simulink model "ZT_VehCtrl_18B"  (R2018b)
settings: Solver=FixedStepAuto  StartTime=0.0  StopTime=inf  FixedStep=0.005  RelTol=1e-3
InitFcn:
  | mbd_mpc_consistency_checks(bdroot(gcs));
undefined symbols (not defined in the file): ANG_DEAD, BMS_NormalPwr, BrkPrsByBrkPct_TB_X, BrkPrsByBrkPct_TB_Y, DELAY_DISCHARGE, DELAY_RCUOFF, DRV_BACKWARD, DRV_BRAKE, DRV_FORWARD, DRV_NEUTRAL, DRV_PARK, DRV_UNPARK, DRV_ZEROTURN, EPB_LOCK, EPB_UNLOCK, ExtraLoadPwr, FanOff, fifo_0_vect, fifo_1_vect, HiFanReq, HV_finished, HV_No_Active, HV_POWER_OFF, HV_POWER_ON, HVDown, HVON, KaTLS_v_DrgUp_X_VehSpd, KeFTM_s_Way1OffDlyTime, KeFTM_TK_Way1CoolLv2OffBatTemp, KeFTM_TK_Way1CoolLv2OffMtrTemp, KeFTM_TK_Way1CoolLv2OnBatTemp, KeFTM_TK_Way1CoolLv2OnMtrTemp, KeFTM_TK_Way1CoolLv3OffBatTemp, KeFTM_TK_Way1CoolLv3OffMtrTemp, KeFTM_TK_Way1CoolLv3OnBatTemp, KeFTM_TK_Way1CoolLv3OnMtrTemp, KeFTM_TK_Way1CoolLv4OffBatTemp, KeFTM_TK_Way1CoolLv4OffMtrTemp, KeFTM_TK_Way1CoolLv4OnBatTemp, KeFTM_TK_Way1CoolLv4OnMtrTemp, Kp1, Kp2, LowFanReq, LQFP, MtrPwrFactor_RCU, MtrPwrHighToMidThd, MtrPwrLowToMidThd, MtrPwrMidToHighThd, MtrPwrMidToLowThd, MtrTrqMax, PCT_DEAD, Precharge, PTO_1000, PTO_540, pts1_fifo_0_vect, pts1_fifo_1_vect, pts2_fifo_0_vect, pts2_fifo_1_vect, pts3_fifo_0_vect, pts3_fifo_1_vect ... (+24)
libraries: mbd_mpc574x_ec_toolbox x124, canmsglib x72, simulink x57
(part 3 of 11)

== system ZT_VehCtrl_18B/SigIn/PWM ==
  note: DI PWM PULLDOWN
  note: DI PWM PULLUP
  Bus Creator : BusCreator  Inputs=8
  Data Store Read : DataStoreRead  DataStoreName=DI31_PWM_DC
  Data Store Read1 : DataStoreRead  DataStoreName=DI31_PWM_FRQ
  Data Store Read2 : DataStoreRead  DataStoreName=DI32_PWM_DC
  Data Store Read3 : DataStoreRead  DataStoreName=DI32_PWM_FRQ
  Data Store Read4 : DataStoreRead  DataStoreName=DI33_PWM_DC
  Data Store Read5 : DataStoreRead  DataStoreName=DI33_PWM_FRQ
  Data Store Read6 : DataStoreRead  DataStoreName=DI34_PWM_DC
  Data Store Read7 : DataStoreRead  DataStoreName=DI34_PWM_FRQ
  Data Store Write : DataStoreWrite  DataStoreName=DI31_PWM_DC
  Data Store Write1 : DataStoreWrite  DataStoreName=DI31_PWM_FRQ
  Data Store Write2 : DataStoreWrite  DataStoreName=DI32_PWM_DC
  Data Store Write3 : DataStoreWrite  DataStoreName=DI32_PWM_FRQ
  Data Store Write4 : DataStoreWrite  DataStoreName=DI33_PWM_DC
  Data Store Write5 : DataStoreWrite  DataStoreName=DI33_PWM_FRQ
  Data Store Write6 : DataStoreWrite  DataStoreName=DI34_PWM_FRQ
  Data Store Write7 : DataStoreWrite  DataStoreName=DI34_PWM_DC
  PWM_PTS1 : Subsystem
  PWM_PTS2 : Subsystem
  PWM_PTS3 : Subsystem
  PWM_PTS4 : Subsystem
  Subsystem : Subsystem  Commented=on
  eTimer_Arm_Capture : mbd_mpc574x_ec_toolbox/Motor Control Blocks/eTIMER Blocks/eTimer_Arm_Capture  etimerModule=0  etimerChannel=2  etimerArmAction=Start
  eTimer_Arm_Capture1 : mbd_mpc574x_ec_toolbox/Motor Control Blocks/eTIMER Blocks/eTimer_Arm_Capture  etimerModule=1  etimerChannel=2  etimerArmAction=Start
  eTimer_Arm_Capture2 : mbd_mpc574x_ec_toolbox/Motor Control Blocks/eTIMER Blocks/eTimer_Arm_Capture  etimerModule=1  etimerChannel=1  etimerArmAction=Start
  eTimer_Arm_Capture3 : mbd_mpc574x_ec_toolbox/Motor Control Blocks/eTIMER Blocks/eTimer_Arm_Capture  etimerModule=1  etimerChannel=3  etimerArmAction=Start
  PWMIn : Outport
  wires:
  Bus Creator/1 -> PWMIn/1
  Data Store Read7/1 -> Bus Creator/8  "DI34_PWM_FRQ"
  Data Store Read6/1 -> Bus Creator/7  "DI34_PWM_DC"
  Data Store Read5/1 -> Bus Creator/6  "DI33_PWM_FRQ"
  Data Store Read4/1 -> Bus Creator/5  "DI33_PWM_DC"
  Data Store Read3/1 -> Bus Creator/4  "DI32_PWM_FRQ"
  Data Store Read2/1 -> Bus Creator/3  "DI32_PWM_DC"
  Data Store Read1/1 -> Bus Creator/2  "DI31_PWM_FRQ"
  Data Store Read/1 -> Bus Creator/1  "DI31_PWM_DC"
  PWM_PTS4/1(DC) -> Data Store Write/1
  PWM_PTS4/2(freq) -> Data Store Write1/1
  PWM_PTS1/1(DC) -> Data Store Write2/1
  PWM_PTS1/2(freq) -> Data Store Write3/1
  PWM_PTS2/1(DC) -> Data Store Write4/1
  PWM_PTS2/2(freq) -> Data Store Write5/1
  PWM_PTS3/2(freq) -> Data Store Write6/1
  PWM_PTS3/1(DC) -> Data Store Write7/1

== system ZT_VehCtrl_18B/SigOut/ACU ==
  "ACU_OUT " : Inport
  Trigger : TriggerPort  VariantControl=Variant  PortDimensions=1
  Bus Selector : BusSelector  OutputSignals=Data,Length
  FCAN_Send_ID_0x0C079AA7 : mbd_mpc574x_ec_toolbox/Communication Blocks/CAN Blocks/FCAN_Send  Priority=2  can_instance=1  can_mode=Non-blocking  can_timeout_ms=0  can_mb_idx=43  can_extended_id=on  can_is_remote=off  can_id=0C079AA7  show_adv_opts=off  can_fd_enable=off  can_enable_brs=off  can_fd_padding=0
      settings: SourceProductName=NXP Model-Based Design Toolbox for MPC57xx MCUs
  VCU_ACU1 : canmsglib/CAN Pack  CANdbFile=D:\VCU\VCU_SL_ZhengZhou\ZT2\模型与接口\CAN_DBC\动力CANB_GBK.dbc  MsgList=VCU_ACU1  MsgName=VCU_ACU1  MsgIDType=Extended (29-bit identifier)  MsgIdentifier=201824935  MsgLength=8  SignalInfo=DcacAcCmd$32$8$1$2$1$0$1$0$-Inf$Inf$#DcacEpsCmd$16$8$1$2$1$0$1$0$-Inf$Inf$#DcacEpsMode$24$8$1$2$1$0$1$0$-Inf$Inf$#DcdcCmd$0$8$1$2$1$0$1$0$-Inf$Inf$#  NSignals=4  StartBits=str2num('[int32(32);int32(16);int32(24);int32(0)]')  SignalSizes=str2num('[int32(8);int32(8);int32(8);int32(8)]')  ByteOrders=str2num('[int32(1);int32(1);int32(1);int32(1)]')  DataTypes=str2num('[int32(2);int32(2);int32(2);int32(2)]')  MultiplexTypes=str2num('[int32(1);int32(1);int32(1);int32(1)]')  MultiplexValues=str2num('[double(0);double(0);double(0);double(0)]')  Factors=str2num('[double(1);double(1);double(1);double(1)]')  Offsets=str2num('[double(0);double(0);double(0);double(0)]')  Minimums=str2num('[double(-Inf);double(-Inf);double(-Inf);double(-Inf)]')  Maximums=str2num('[double(Inf);double(Inf);double(Inf);double(Inf)]')  Remote=off  ApplyMinMax=off  BusOutput=on
      settings: SourceProductName=Simulink Real-Time  SourceProductBaseCode=XP  DataFormat=CANdb specified signals
  wires:
  VCU_ACU1/1 -> Bus Selector/1
  Bus Selector/2 -> FCAN_Send_ID_0x0C079AA7/2  "<Length>"
  Bus Selector/1 -> FCAN_Send_ID_0x0C079AA7/1  "<Data>"

== system ZT_VehCtrl_18B/SigOut/BMS ==
  "BMS_OUT " : Inport
  Trigger : TriggerPort  VariantControl=Variant  PortDimensions=1
  Bus Selector : BusSelector  OutputSignals=Data,Length
  FCAN_Send_ID_0x160 : mbd_mpc574x_ec_toolbox/Communication Blocks/CAN Blocks/FCAN_Send  Priority=2  can_instance=0  can_mode=Non-blocking  can_timeout_ms=0  can_mb_idx=43  can_extended_id=off  can_is_remote=off  can_id=160  show_adv_opts=off  can_fd_enable=off  can_enable_brs=off  can_fd_padding=0
      settings: SourceProductName=NXP Model-Based Design Toolbox for MPC57xx MCUs
  VCU_BMS : canmsglib/CAN Pack  CANdbFile=D:\VCU\VCU_SL_ZhengZhou\ZT2\模型与接口\CAN_DBC\整车CANA_GBK.dbc  MsgList=VCU_BMS  MsgName=VCU_BMS  MsgIDType=Standard (11-bit identifier)  MsgIdentifier=352  MsgLength=8  SignalInfo=VCU_PowerOnReq$0$1$2$2$1$0$1$0$0$1$#VCU_UrgencyCutOffPowerReq$1$1$2$2$1$0$1$0$0$1$#  NSignals=2  StartBits=str2num('[int32(0);int32(1)]')  SignalSizes=str2num('[int32(1);int32(1)]')  ByteOrders=str2num('[int32(2);int32(2)]')  DataTypes=str2num('[int32(2);int32(2)]')  MultiplexTypes=str2num('[int32(1);int32(1)]')  MultiplexValues=str2num('[double(0);double(0)]')  Factors=str2num('[double(1);double(1)]')  Offsets=str2num('[double(0);double(0)]')  Minimums=str2num('[double(0);double(0)]')  Maximums=str2num('[double(1);double(1)]')  Remote=off  ApplyMinMax=off  BusOutput=on
      settings: SourceProductName=Simulink Real-Time  SourceProductBaseCode=XP  DataFormat=CANdb specified signals
  wires:
  VCU_BMS/1 -> Bus Selector/1
  Bus Selector/2 -> FCAN_Send_ID_0x160/2  "<Length>"
  Bus Selector/1 -> FCAN_Send_ID_0x160/1  "<Data>"

== system ZT_VehCtrl_18B/SigOut/BRS ==
  "BRS_OUT " : Inport
  Trigger : TriggerPort  VariantControl=Variant  PortDimensions=1
  Bus Selector : BusSelector  OutputSignals=Data,Length
  Bus Selector1 : BusSelector  OutputSignals=DCDC_Enable
  FCAN_Send_ID_0x0CF109A7 : mbd_mpc574x_ec_toolbox/Communication Blocks/CAN Blocks/FCAN_Send  Priority=2  can_instance=0  can_mode=Non-blocking  can_timeout_ms=0  can_mb_idx=44  can_extended_id=on  can_is_remote=off  can_id=0CF109A7  show_adv_opts=off  can_fd_enable=off  can_enable_brs=off  can_fd_padding=0
      settings: SourceProductName=NXP Model-Based Design Toolbox for MPC57xx MCUs
  VCU2BRS : canmsglib/CAN Pack  CANdbFile=D:\VCU\VCU_SL_ZhengZhou\ZT2\模型与接口\CAN_DBC\整车CANA_GBK.dbc  MsgList=VCU2BRS  MsgName=VCU2BRS  MsgIDType=Extended (29-bit identifier)  MsgIdentifier=217123239  MsgLength=8  SignalInfo=LiveCounter$56$8$1$2$1$0$1$0$0$255$#MaxChargePowerLimit$16$16$1$2$1$0$1$0$0$500$#OnOffCmd$46$1$1$2$1$0$1$0$0$1$#PowerReq$0$16$1$2$1$0$1$0$0$500$#  NSignals=4  StartBits=str2num('[int32(56);int32(16);int32(46);int32(0)]')  SignalSizes=str2num('[int32(8);int32(16);int32(1);int32(16)]')  ByteOrders=str2num('[int32(1);int32(1);int32(1);int32(1)]')  DataTypes=str2num('[int32(2);int32(2);int32(2);int32(2)]')  MultiplexTypes=str2num('[int32(1);int32(1);int32(1);int32(1)]')  MultiplexValues=str2num('[double(0);double(0);double(0);double(0)]')  Factors=str2num('[double(1);double(1);double(1);double(1)]')  Offsets=str2num('[double(0);double(0);double(0);double(0)]')  Minimums=str2num('[double(0);double(0);double(0);double(0)]')  Maximums=str2num('[double(255);double(500);double(1);double(500)]')  Remote=off  ApplyMinMax=off  BusOutput=on
      settings: SourceProductName=Simulink Real-Time  SourceProductBaseCode=XP  DataFormat=CANdb specified signals
  wires:
  VCU2BRS/1 -> Bus Selector/1
  "BRS_OUT "/1 -> Bus Selector1/1
  Bus Selector/1 -> FCAN_Send_ID_0x0CF109A7/1  "<Data>"
  Bus Selector/2 -> FCAN_Send_ID_0x0CF109A7/2  "<Length>"

== system ZT_VehCtrl_18B/SigOut/DCDC ==
  "DCDC_OUT " : Inport
  Trigger : TriggerPort  VariantControl=Variant  PortDimensions=1
  Bus Selector : BusSelector  OutputSignals=Data,Length
  FCAN_Send_ID_0x18008FD0 : mbd_mpc574x_ec_toolbox/Communication Blocks/CAN Blocks/FCAN_Send  Priority=2  can_instance=1  can_mode=Non-blocking  can_timeout_ms=0  can_mb_idx=43  can_extended_id=on  can_is_remote=off  can_id=18008FD0  show_adv_opts=off  can_fd_enable=off  can_enable_brs=off  can_fd_padding=0
      settings: SourceProductName=NXP Model-Based Design Toolbox for MPC57xx MCUs
  VCU_DCDC1 : canmsglib/CAN Pack  CANdbFile=D:\VCU\VCU_SL_ZhengZhou\ZT2\模型与接口\CAN_DBC\动力CANB_GBK.dbc  MsgList=VCU_DCDC1  MsgName=VCU_DCDC1  MsgIDType=Extended (29-bit identifier)  MsgIdentifier=402690000  MsgLength=8  SignalInfo=VCU_DCDC1_En$0$2$1$2$1$0$1$0$0$3$#  NSignals=1  StartBits=str2num('[int32(0)]')  SignalSizes=str2num('[int32(2)]')  ByteOrders=str2num('[int32(1)]')  DataTypes=str2num('[int32(2)]')  MultiplexTypes=str2num('[int32(1)]')  MultiplexValues=str2num('[double(0)]')  Factors=str2num('[double(1)]')  Offsets=str2num('[double(0)]')  Minimums=str2num('[double(0)]')  Maximums=str2num('[double(3)]')  Remote=off  ApplyMinMax=off  BusOutput=on
      settings: SourceProductName=Simulink Real-Time  SourceProductBaseCode=XP  DataFormat=CANdb specified signals
  wires:
  VCU_DCDC1/1 -> Bus Selector/1
  Bus Selector/2 -> FCAN_Send_ID_0x18008FD0/2  "<Length>"
  Bus Selector/1 -> FCAN_Send_ID_0x18008FD0/1  "<Data>"

== system ZT_VehCtrl_18B/SigOut/GPIO  ==
  note: LS
  note: PWM
  note: HS
  ETC : Subsystem
  HS : Subsystem
  PWM_OUT : Subsystem  Commented=on
  SPI0: LS09_14_15_16_1_2_11_4 : Subsystem
  SPI3: LS03_06_07_08_10_12_13_17_18_19 : Subsystem

== system ZT_VehCtrl_18B/SigOut/HVC ==
  "HVC_OUT " : Inport
  Trigger : TriggerPort  VariantControl=Variant  PortDimensions=1
  Bus Selector : BusSelector  OutputSignals=Data,Length
  Ctrl_HVC : canmsglib/CAN Pack  CANdbFile=D:\VCU\VCU_SL_ZhengZhou\ZT2\模型与接口\CAN_DBC\动力CANB_GBK.dbc  MsgList=Ctrl_HVC  MsgName=Ctrl_HVC  MsgIDType=Extended (29-bit identifier)  MsgIdentifier=402694405  MsgLength=8  SignalInfo=EDrv1_PowOnCmd$0$1$1$2$1$0$1$0$0$1$#EDrv2_PowOnCmd$2$1$1$2$1$0$1$0$0$1$#HvcCmd_Life$60$4$1$2$1$0$1$0$0$15$#PTC_PowOnCmd$6$1$1$2$1$0$1$0$0$1$#PaxAC_PowOnCmd$4$1$1$2$1$0$1$0$0$1$#  NSignals=5  StartBits=str2num('[int32(0);int32(2);int32(60);int32(6);int32(4)]')  SignalSizes=str2num('[int32(1);int32(1);int32(4);int32(1);int32(1)]')  ByteOrders=str2num('[int32(1);int32(1);int32(1);int32(1);int32(1)]')  DataTypes=str2num('[int32(2);int32(2);int32(2);int32(2);int32(2)]')  MultiplexTypes=str2num('[int32(1);int32(1);int32(1);int32(1);int32(1)]')  MultiplexValues=str2num('[double(0);double(0);double(0);double(0);double(0)]')  Factors=str2num('[double(1);double(1);double(1);double(1);double(1)]')  Offsets=str2num('[double(0);double(0);double(0);double(0);double(0)]')  Minimums=str2num('[double(0);double(0);double(0);double(0);double(0)]')  Maximums=str2num('[double(1);double(1);double(15);double(1);double(1)]')  Remote=off  ApplyMinMax=off  BusOutput=on
      settings: SourceProductName=Simulink Real-Time  SourceProductBaseCode=XP  DataFormat=CANdb specified signals
  FCAN_Send_ID_0x1800A105 : mbd_mpc574x_ec_toolbox/Communication Blocks/CAN Blocks/FCAN_Send  Priority=2  can_instance=1  can_mode=Non-blocking  can_timeout_ms=0  can_mb_idx=43  can_extended_id=on  can_is_remote=off  can_id=1800A105  show_adv_opts=off  can_fd_enable=off  can_enable_brs=off  can_fd_padding=0
      settings: SourceProductName=NXP Model-Based Design Toolbox for MPC57xx MCUs
  wires:
  Bus Selector/1 -> FCAN_Send_ID_0x1800A105/1  "<Data>"
  Bus Selector/2 -> FCAN_Send_ID_0x1800A105/2  "<Length>"
  Ctrl_HVC/1 -> Bus Selector/1

== system ZT_VehCtrl_18B/SigOut/ICU1  ==
  "ICU_OUT " : Inport
  Trigger : TriggerPort  VariantControl=Variant  PortDimensions=1
  Bus Selector{,3..7} (6 alike) : BusSelector  OutputSignals=Data,Length
  Bus Selector1 : BusSelector  OutputSignals=DCDC_Enable
  FCAN_Send_ID_0x180128D0 : mbd_mpc574x_ec_toolbox/Communication Blocks/CAN Blocks/FCAN_Send  Priority=2  can_instance=0  can_mode=Non-blocking  can_timeout_ms=0  can_mb_idx=44  can_extended_id=on  can_is_remote=off  can_id=180128D0  show_adv_opts=off  can_fd_enable=off  can_enable_brs=off  can_fd_padding=0
      settings: SourceProductName=NXP Model-Based Design Toolbox for MPC57xx MCUs
  FCAN_Send_ID_0x180328D0 : mbd_mpc574x_ec_toolbox/Communication Blocks/CAN Blocks/FCAN_Send  Priority=2  can_instance=0  can_mode=Non-blocking  can_timeout_ms=0  can_mb_idx=44  can_extended_id=on  can_is_remote=off  can_id=180328D0  show_adv_opts=off  can_fd_enable=off  can_enable_brs=off  can_fd_padding=0
      settings: SourceProductName=NXP Model-Based Design Toolbox for MPC57xx MCUs
  FCAN_Send_ID_0x181128D0 : mbd_mpc574x_ec_toolbox/Communication Blocks/CAN Blocks/FCAN_Send  Priority=2  can_instance=0  can_mode=Non-blocking  can_timeout_ms=0  can_mb_idx=44  can_extended_id=on  can_is_remote=off  can_id=181128D0  show_adv_opts=off  can_fd_enable=off  can_enable_brs=off  can_fd_padding=0
      settings: SourceProductName=NXP Model-Based Design Toolbox for MPC57xx MCUs
  FCAN_Send_ID_0x181228D0 : mbd_mpc574x_ec_toolbox/Communication Blocks/CAN Blocks/FCAN_Send  Priority=2  can_instance=0  can_mode=Non-blocking  can_timeout_ms=0  can_mb_idx=44  can_extended_id=on  can_is_remote=off  can_id=181228D0  show_adv_opts=off  can_fd_enable=off  can_enable_brs=off  can_fd_padding=0
      settings: SourceProductName=NXP Model-Based Design Toolbox for MPC57xx MCUs
  FCAN_Send_ID_0x181328D0 : mbd_mpc574x_ec_toolbox/Communication Blocks/CAN Blocks/FCAN_Send  Priority=2  can_instance=1  can_mode=Non-blocking  can_timeout_ms=0  can_mb_idx=44  can_extended_id=on  can_is_remote=off  can_id=181328D0  show_adv_opts=off  can_fd_enable=off  can_enable_brs=off  can_fd_padding=0
      settings: SourceProductName=NXP Model-Based Design Toolbox for MPC57xx MCUs
  FCAN_Send_ID_0x181428D0 : mbd_mpc574x_ec_toolbox/Communication Blocks/CAN Blocks/FCAN_Send  Priority=2  can_instance=1  can_mode=Non-blocking  can_timeout_ms=0  can_mb_idx=44  can_extended_id=on  can_is_remote=off  can_id=181428D0  show_adv_opts=off  can_fd_enable=off  can_enable_brs=off  can_fd_padding=0
      settings: SourceProductName=NXP Model-Based Design Toolbox for MPC57xx MCUs
  VCU2MCU1_1 : canmsglib/CAN Pack  CANdbFile=D:\VCU\VCU_SL_ZhengZhou\ZT2\模型与接口\CAN_DBC\整车CANA_GBK.dbc  MsgList=VCU2ICUInfor1  MsgName=VCU2ICUInfor1  MsgIDType=Extended (29-bit identifier)  MsgIdentifier=402729168  MsgLength=8  SignalInfo=VCU_BattSOC_pct$16$8$1$2$1$0$1$0$0$100$#VCU_BattTempHi_b$32$1$1$2$1$0$1$0$0$1$#VCU_BrakeFlt_b$39$1$1$2$1$0$1$0$0$1$#VCU_CoolFanWrkIdc_b$44$1$1$2$1$0$1$0$0$1$#VCU_CoolSysFanPWM$56$8$1$2$1$0$1$0$0$100$#VCU_CoolSysFltIdc_b$43$1$1$2$1$0$1$0$0$1$#VCU_EmrPumpSt_enum$5$2$1$2$1$0$1$0$0$3$#VCU_FltSt_enum$6$1$1$2$1$0$1$0$0$1$#VCU_GearSt_enum$24$8$1$2$1$0$1$0$0$5$#VCU_HeadLight_b$46$1$1$2$1$0$1$0$0$1$#VCU_HydSysFlt_b$33$1$1$2$1$0$1$0$0$1$#VCU_LShift_b$3$1$1$2$1$0$1$0$0$1$#VCU_MCUTempHiFlt_b$35$1$1$2$1$0$1$0$0$1$#VCU_MtTempHiFlt_b$36$1$1$2$1$0$1$0$0$1$#VCU_Pst_b$0$1$1$2$1$0$1$0$0$1$#VCU_RShift_b$2$1$1$2$1$0$1$0$0$1$#VCU_RearLight_b$45$1$1$2$1$0$1$0$0$1$#VCU_SOCLoFlt_b$1$1$1$2$1$0$1$0$0$1$#VCU_SysWorkStCode_num$48$8$1$2$1$0$1$0$0$255$#VCU_TopWrkSt_b$38$1$1$2$1$0$1$0$0$1$#VCU_VehACharge_b$34$1$1$2$1$0$1$0$0$1$#VCU_VehDCharge_b$37$1$1$2$1$0$1$0$0$1$#VCU_VehSpd_kmh$8$8$1$2$1$0$1$0$0$255$#VCU_WatPumpOpenSt_b$47$1$1$2$1$0$1$0$0$1$#VCU_WrkSt_enum$7$1$1$2$1$0$1$0$0$1$#  NSignals=25  StartBits=str2num('[int32(16);int32(32);int32(39);int32(44);int32(56);int32(43);int32(5);int32(6);int32(24);int32(46);int32(33);int32(3);int32(35);int32(36);int32(0);int32(2);int32(45);int32(1);int32(48);int32(38);int32(34);int32(37);int32(8);int32(47);int32(7)]')  SignalSizes=str2num('[int32(8);int32(1);int32(1);int32(1);int32(8);int32(1);int32(2);int32(1);int32(8);int32(1);int32(1);int32(1);int32(1);int32(1);int32(1);int32(1);int32(1);int32(1);int32(8);int32(1);int32(1);int32(1);int32(8);int32(1);int32(1)]')  ByteOrders=str2num('[int32(1);int32(1);int32(1);int32(1);int32(1);int32(1);int32(1);int32(1);int32(1);int32(1);int32(1);int32(1);int32(1);int32(1);int32(1);int32(1);int32(1);int32(1);int32(1);int32(1);int32(1);int32(1);int32(1);int32(1);int32(1)]')  DataTypes=str2num('[int32(2);int32(2);int32(2);int32(2);int32(2);int32(2);int32(2);int32(2);int32(2);int32(2);int32(2);int32(2);int32(2);int32(2);int32(2);int32(2);int32(2);int32(2);int32(2);int32(2);int32(2);int32(2);int32(2);int32(2);int32(2)]')  MultiplexTypes=str2num('[int32(1);int32(1);int32(1);int32(1);int32(1);int32(1);int32(1);int32(1);int32(1);int32(1);int32(1);int32(1);int32(1);int32(1);int32(1);int32(1);int32(1);int32(1);int32(1);int32(1);int32(1);int32(1);int32(1);int32(1);int32(1)]')  MultiplexValues=str2num('[double(0);double(0);double(0);double(0);double(0);double(0);double(0);double(0);double(0);double(0);double(0);double(0);double(0);double(0);double(0);double(0);double(0);double(0);double(0);double(0);double(0);double(0);double(0);double(0);double(0)]')  Factors=str2num('[double(1);double(1);double(1);double(1);double(1);double(1);double(1);double(1);double(1);double(1);double(1);double(1);double(1);double(1);double(1);double(1);double(1);double(1);double(1);double(1);double(1);double(1);double(1);double(1);double(1)]')  Offsets=str2num('[double(0);double(0);double(0);double(0);double(0);double(0);double(0);double(0);double(0);double(0);double(0);double(0);double(0);double(0);double(0);double(0);double(0);double(0);double(0);double(0);double(0);double(0);double(0);double(0);double(0)]')  Minimums=str2num('[double(0);double(0);double(0);double(0);double(0);double(0);double(0);double(0);double(0);double(0);double(0);double(0);double(0);double(0);double(0);double(0);double(0);double(0);double(0);double(0);double(0);double(0);double(0);double(0);double(0)]')  Maximums=str2num('[double(100);double(1);double(1);double(1);double(100);double(1);double(3);double(1);double(5);double(1);double(1);double(1);double(1);double(1);double(1);double(1);double(1);double(1);double(255);double(1);double(1);double(1);double(255);double(1);double(1)]')  Remote=off  ApplyMinMax=off  BusOutput=on
      settings: SourceProductName=Simulink Real-Time  SourceProductBaseCode=XP  DataFormat=CANdb specified signals
  VCU2MCU1_3 : canmsglib/CAN Pack  CANdbFile=D:\VCU\VCU_SL_ZhengZhou\ZT2\模型与接口\CAN_DBC\整车CANA_GBK.dbc  MsgList=VCU2ICUInfor3  MsgName=VCU2ICUInfor3  MsgIDType=Extended (29-bit identifier)  MsgIdentifier=402860240  MsgLength=8  SignalInfo=VCU_BattBusVolt_V$48$16$1$2$1$0$1.000000e-01$0$0$6.553500e+03$#VCU_EVFltCode1_num$24$8$1$2$1$0$1$0$0$255$#VCU_EVFltCode2_num$32$8$1$2$1$0$1$0$0$255$#VCU_EVFltLvlMax_num$40$8$1$2$1$0$1$0$0$3$#VCU_HistFltCode1_num$0$8$1$2$1$0$1$0$0$255$#VCU_HistFltCode2_num$8$8$1$2$1$0$1$0$0$255$#VCU_HistFltCode3_num$16$8$1$2$1$0$1$0$0$255$#  NSignals=7  StartBits=str2num('[int32(48);int32(24);int32(32);int32(40);int32(0);int32(8);int32(16)]')  SignalSizes=str2num('[int32(16);int32(8);int32(8);int32(8);int32(8);int32(8);int32(8)]')  ByteOrders=str2num('[int32(1);int32(1);int32(1);int32(1);int32(1);int32(1);int32(1)]')  DataTypes=str2num('[int32(2);int32(2);int32(2);int32(2);int32(2);int32(2);int32(2)]')  MultiplexTypes=str2num('[int32(1);int32(1);int32(1);int32(1);int32(1);int32(1);int32(1)]')  MultiplexValues=str2num('[double(0);double(0);double(0);double(0);double(0);double(0);double(0)]')  Factors=str2num('[double(1.000000e-01);double(1);double(1);double(1);double(1);double(1);double(1)]')  Offsets=str2num('[double(0);double(0);double(0);double(0);double(0);double(0);double(0)]')  Minimums=str2num('[double(0);double(0);double(0);double(0);double(0);double(0);double(0)]')  Maximums=str2num('[double(6.553500e+03);double(255);double(255);double(3);double(255);double(255);double(255)]')  Remote=off  ApplyMinMax=off  BusOutput=on
      settings: SourceProductName=Simulink Real-Time  SourceProductBaseCode=XP  DataFormat=CANdb specified signals
  VCU2MCU1_4 : canmsglib/CAN Pack  CANdbFile=D:\VCU\VCU_SL_ZhengZhou\ZT2\模型与接口\CAN_DBC\整车CANA_GBK.dbc  MsgList=VCU2ICUInfor4  MsgName=VCU2ICUInfor4  MsgIDType=Extended (29-bit identifier)  MsgIdentifier=403777744  MsgLength=8  SignalInfo=VCU_BattTempMax_deg$48$8$1$1$1$0$1$-40$-40$215$#VCU_BattTempMin_deg$40$8$1$1$1$0$1$-40$-40$215$#VCU_CoolWaterTemp_deg$16$8$1$1$1$0$1$-40$-40$215$#VCU_DrvMtCtlUnitTemp_deg$32$8$1$1$1$0$1$-40$-40$215$#VCU_DrvMtTemp_deg$24$8$1$1$1$0$1$-40$-40$215$#VCU_OilMtCtlUnitTemp_deg$8$8$1$1$1$0$1$-40$-40$215$#VCU_OilMtTemp_deg$0$8$1$1$1$0$1$-40$-40$215$#VCU_RemindInfor_num$56$8$1$2$1$0$1$0$-Inf$Inf$#  NSignals=8  StartBits=str2num('[int32(48);int32(40);int32(16);int32(32);int32(24);int32(8);int32(0);int32(56)]')  SignalSizes=str2num('[int32(8);int32(8);int32(8);int32(8);int32(8);int32(8);int32(8);int32(8)]')  ByteOrders=str2num('[int32(1);int32(1);int32(1);int32(1);int32(1);int32(1);int32(1);int32(1)]')  DataTypes=str2num('[int32(1);int32(1);int32(1);int32(1);int32(1);int32(1);int32(1);int32(2)]')  MultiplexTypes=str2num('[int32(1);int32(1);int32(1);int32(1);int32(1);int32(1);int32(1);int32(1)]')  MultiplexValues=str2num('[double(0);double(0);double(0);double(0);double(0);double(0);double(0);double(0)]')  Factors=str2num('[double(1);double(1);double(1);double(1);double(1);double(1);double(1);double(1)]')  Offsets=str2num('[double(-40);double(-40);double(-40);double(-40);double(-40);double(-40);double(-40);double(0)]')  Minimums=str2num('[double(-40);double(-40);double(-40);double(-40);double(-40);double(-40);double(-40);double(-Inf)]')  Maximums=str2num('[double(215);double(215);double(215);double(215);double(215);double(215);double(215);double(Inf)]')  Remote=off  ApplyMinMax=off  BusOutput=on
      settings: SourceProductName=Simulink Real-Time  SourceProductBaseCode=XP  DataFormat=CANdb specified signals
  VCU2MCU1_5 : canmsglib/CAN Pack  CANdbFile=D:\VCU\VCU_SL_ZhengZhou\ZT2\模型与接口\CAN_DBC\整车CANA_GBK.dbc  MsgList=VCU2ICUInfor5  MsgName=VCU2ICUInfor5  MsgIDType=Extended (29-bit identifier)  MsgIdentifier=403843280  MsgLength=8  SignalInfo=VCU_DrvMCUBusCurr_A$48$16$1$1$1$0$1$-1000$-1000$35535$#VCU_DrvMCUBusVolt_V$32$16$1$2$1$0$1$0$0$65535$#VCU_DrvMtSpd_rpm$0$16$1$1$1$0$1$-30000$-30000$35535$#VCU_DrvMtTrq_Nm$16$16$1$2$1$0$1$0$0$65535$#  NSignals=4  StartBits=str2num('[int32(48);int32(32);int32(0);int32(16)]')  SignalSizes=str2num('[int32(16);int32(16);int32(16);int32(16)]')  ByteOrders=str2num('[int32(1);int32(1);int32(1);int32(1)]')  DataTypes=str2num('[int32(1);int32(2);int32(1);int32(2)]')  MultiplexTypes=str2num('[int32(1);int32(1);int32(1);int32(1)]')  MultiplexValues=str2num('[double(0);double(0);double(0);double(0)]')  Factors=str2num('[double(1);double(1);double(1);double(1)]')  Offsets=str2num('[double(-1000);double(0);double(-30000);double(0)]')  Minimums=str2num('[double(-1000);double(0);double(-30000);double(0)]')  Maximums=str2num('[double(35535);double(65535);double(35535);double(65535)]')  Remote=off  ApplyMinMax=off  BusOutput=on
      settings: SourceProductName=Simulink Real-Time  SourceProductBaseCode=XP  DataFormat=CANdb specified signals
  VCU2MCU1_6 : canmsglib/CAN Pack  CANdbFile=D:\VCU\VCU_SL_ZhengZhou\ZT2\模型与接口\CAN_DBC\整车CANA_GBK.dbc  MsgList=VCU2ICUInfor6  MsgName=VCU2ICUInfor6  MsgIDType=Extended (29-bit identifier)  MsgIdentifier=403908816  MsgLength=8  SignalInfo=VCU_OilMCUBusCurr_A$48$16$1$1$1$0$1$-1000$-1000$35535$#VCU_OilMCUBusVolt_V$32$16$1$2$1$0$1$0$0$65535$#VCU_OilMtSpd_rpm$0$16$1$2$1$0$1$0$0$65535$#VCU_OilMtTrq_Nm$16$16$1$2$1$0$1$0$0$65535$#  NSignals=4  StartBits=str2num('[int32(48);int32(32);int32(0);int32(16)]')  SignalSizes=str2num('[int32(16);int32(16);int32(16);int32(16)]')  ByteOrders=str2num('[int32(1);int32(1);int32(1);int32(1)]')  DataTypes=str2num('[int32(1);int32(2);int32(2);int32(2)]')  MultiplexTypes=str2num('[int32(1);int32(1);int32(1);int32(1)]')  MultiplexValues=str2num('[double(0);double(0);double(0);double(0)]')  Factors=str2num('[double(1);double(1);double(1);double(1)]')  Offsets=str2num('[double(-1000);double(0);double(0);double(0)]')  Minimums=str2num('[double(-1000);double(0);double(0);double(0)]')  Maximums=str2num('[double(35535);double(65535);double(65535);double(65535)]')  Remote=off  ApplyMinMax=off  BusOutput=on
      settings: SourceProductName=Simulink Real-Time  SourceProductBaseCode=XP  DataFormat=CANdb specified signals
  VCU2MCU1_7 : canmsglib/CAN Pack  CANdbFile=D:\VCU\VCU_SL_ZhengZhou\ZT2\模型与接口\CAN_DBC\整车CANA_GBK.dbc  MsgList=VCU2ICUInfor7  MsgName=VCU2ICUInfor7  MsgIDType=Extended (29-bit identifier)  MsgIdentifier=403974352  MsgLength=8  SignalInfo=VCU_DisChargePwr_kw$0$16$1$2$1$0$1.000000e-01$0$0$10000$#VCU_RangeRemain_km$48$16$1$2$1$0$1$0$0$65535$#VCU_RegenPwr_kw$16$16$1$2$1$0$1.000000e-01$0$0$10000$#VCU_RunAllMile_km$32$16$1$2$1$0$1$0$0$65535$#  NSignals=4  StartBits=str2num('[int32(0);int32(48);int32(16);int32(32)]')  SignalSizes=str2num('[int32(16);int32(16);int32(16);int32(16)]')  ByteOrders=str2num('[int32(1);int32(1);int32(1);int32(1)]')  DataTypes=str2num('[int32(2);int32(2);int32(2);int32(2)]')  MultiplexTypes=str2num('[int32(1);int32(1);int32(1);int32(1)]')  MultiplexValues=str2num('[double(0);double(0);double(0);double(0)]')  Factors=str2num('[double(1.000000e-01);double(1);double(1.000000e-01);double(1)]')  Offsets=str2num('[double(0);double(0);double(0);double(0)]')  Minimums=str2num('[double(0);double(0);double(0);double(0)]')  Maximums=str2num('[double(10000);double(65535);double(10000);double(65535)]')  Remote=off  ApplyMinMax=off  BusOutput=on
      settings: SourceProductName=Simulink Real-Time  SourceProductBaseCode=XP  DataFormat=CANdb specified signals
  wires:
  VCU2MCU1_1/1 -> Bus Selector/1
  "ICU_OUT "/1 -> Bus Selector1/1
  Bus Selector/1 -> FCAN_Send_ID_0x180128D0/1  "<Data>"
  Bus Selector/2 -> FCAN_Send_ID_0x180128D0/2  "<Length>"
  VCU2MCU1_3/1 -> Bus Selector3/1
  Bus Selector3/1 -> FCAN_Send_ID_0x180328D0/1  "<Data>"
  Bus Selector3/2 -> FCAN_Send_ID_0x180328D0/2  "<Length>"
  Bus Selector4/2 -> FCAN_Send_ID_0x181128D0/2  "<Length>"
  Bus Selector4/1 -> FCAN_Send_ID_0x181128D0/1  "<Data>"
  VCU2MCU1_4/1 -> Bus Selector4/1
  VCU2MCU1_5/1 -> Bus Selector5/1
  Bus Selector5/1 -> FCAN_Send_ID_0x181228D0/1  "<Data>"
  Bus Selector5/2 -> FCAN_Send_ID_0x181228D0/2  "<Length>"
  Bus Selector6/2 -> FCAN_Send_ID_0x181328D0/2  "<Length>"
  Bus Selector6/1 -> FCAN_Send_ID_0x181328D0/1  "<Data>"
  VCU2MCU1_6/1 -> Bus Selector6/1
  VCU2MCU1_7/1 -> Bus Selector7/1
  Bus Selector7/1 -> FCAN_Send_ID_0x181428D0/1  "<Data>"
  Bus Selector7/2 -> FCAN_Send_ID_0x181428D0/2  "<Length>"

== system ZT_VehCtrl_18B/SigOut/ICU2 ==
  "ICU_OUT " : Inport
  Trigger : TriggerPort  VariantControl=Variant  PortDimensions=1
  Bus Selector : BusSelector  OutputSignals=Data,Length
  FCAN_Send_ID_0x180228D0 : mbd_mpc574x_ec_toolbox/Communication Blocks/CAN Blocks/FCAN_Send  Priority=2  can_instance=0  can_mode=Non-blocking  can_timeout_ms=0  can_mb_idx=45  can_extended_id=on  can_is_remote=off  can_id=180228D0  show_adv_opts=off  can_fd_enable=off  can_enable_brs=off  can_fd_padding=0
      settings: SourceProductName=NXP Model-Based Design Toolbox for MPC57xx MCUs
  VCU2ICUInfor2 : canmsglib/CAN Pack  CANdbFile=D:\VCU\VCU_SL_ZhengZhou\ZT2\模型与接口\CAN_DBC\整车CANA_GBK.dbc  MsgList=VCU2ICUInfor2  MsgName=VCU2ICUInfor2  MsgIDType=Extended (29-bit identifier)  MsgIdentifier=402794704  MsgLength=8  SignalInfo=VCU_AccPedSt_pct$24$8$1$2$1$0$1$0$0$100$#VCU_BattBusCurr_A$8$16$1$1$1$0$1.000000e-01$-1000$-1000$-1000$#VCU_BrakePedSt_pct$32$8$1$2$1$0$1$0$0$100$#VCU_SwVersion_num$0$8$1$2$1$0$1.000000e-01$0$0$255$#VCU_WrkTimeAll_h$40$16$1$2$1$0$1$0$0$65535$#VCU_WrkTimeAll_min$56$8$1$2$1$0$1$0$0$255$#  NSignals=6  StartBits=str2num('[int32(24);int32(8);int32(32);int32(0);int32(40);int32(56)]')  SignalSizes=str2num('[int32(8);int32(16);int32(8);int32(8);int32(16);int32(8)]')  ByteOrders=str2num('[int32(1);int32(1);int32(1);int32(1);int32(1);int32(1)]')  DataTypes=str2num('[int32(2);int32(1);int32(2);int32(2);int32(2);int32(2)]')  MultiplexTypes=str2num('[int32(1);int32(1);int32(1);int32(1);int32(1);int32(1)]')  MultiplexValues=str2num('[double(0);double(0);double(0);double(0);double(0);double(0)]')  Factors=str2num('[double(1);double(1.000000e-01);double(1);double(1.000000e-01);double(1);double(1)]')  Offsets=str2num('[double(0);double(-1000);double(0);double(0);double(0);double(0)]')  Minimums=str2num('[double(0);double(-1000);double(0);double(0);double(0);double(0)]')  Maximums=str2num('[double(100);double(-1000);double(100);double(255);double(65535);double(255)]')  Remote=off  ApplyMinMax=off  BusOutput=on
      settings: SourceProductName=Simulink Real-Time  SourceProductBaseCode=XP  DataFormat=CANdb specified signals
  wires:
  Bus Selector/2 -> FCAN_Send_ID_0x180228D0/2  "<Length>"
  Bus Selector/1 -> FCAN_Send_ID_0x180228D0/1  "<Data>"
  VCU2ICUInfor2/1 -> Bus Selector/1

== system ZT_VehCtrl_18B/SigOut/ISG ==
  "ISG_OUT " : Inport
  Trigger : TriggerPort  VariantControl=Variant  PortDimensions=1
  Bus Selector : BusSelector  OutputSignals=Data,Length
  FCAN_Send_ID_0xCFF06EF : mbd_mpc574x_ec_toolbox/Communication Blocks/CAN Blocks/FCAN_Send  Priority=2  can_instance=1  can_mode=Non-blocking  can_timeout_ms=0  can_mb_idx=43  can_extended_id=on  can_is_remote=off  can_id=CFF06EF  show_adv_opts=off  can_fd_enable=off  can_enable_brs=off  can_fd_padding=0
      settings: SourceProductName=NXP Model-Based Design Toolbox for MPC57xx MCUs
  ISG HCU Command : canmsglib/CAN Pack  CANdbFile=D:\VCU\VCU_SL_ZhengZhou\ZT2\模型与接口\CAN_DBC\动力CANB_GBK.dbc  MsgList=ISG_HCU_Command  MsgName=ISG_HCU_Command  MsgIDType=Extended (29-bit identifier)  MsgIdentifier=218040047  MsgLength=8  SignalInfo=Control_Mode$2$2$1$2$1$0$1$0$-Inf$Inf$#Demand_Limit_High_Positive_Value$8$12$1$2$1$0$4$0$0$16384$#Demand_Limit_Low_Negative_Value$20$12$1$2$1$0$4$0$0$16384$#Demand_Speed$48$16$1$2$1$0$1$-15000$-15000$15000$#Demand_Torque$32$16$1$2$1$0$1$-5000$-5000$5000$#Fault_Reset$1$1$1$2$1$0$1$0$-Inf$Inf$#FootBrake$6$1$1$2$1$0$1$0$-Inf$Inf$#Gear$4$2$1$2$1$0$1$0$-Inf$Inf$#HandBrake$7$1$1$2$1$0$1$0$-Inf$Inf$#MCU_Enable$0$1$1$2$1$0$1$0$-Inf$Inf$#  NSignals=10  StartBits=str2num('[int32(2);int32(8);int32(20);int32(48);int32(32);int32(1);int32(6);int32(4);int32(7);int32(0)]')  SignalSizes=str2num('[int32(2);int32(12);int32(12);int32(16);int32(16);int32(1);int32(1);int32(2);int32(1);int32(1)]')  ByteOrders=str2num('[int32(1);int32(1);int32(1);int32(1);int32(1);int32(1);int32(1);int32(1);int32(1);int32(1)]')  DataTypes=str2num('[int32(2);int32(2);int32(2);int32(2);int32(2);int32(2);int32(2);int32(2);int32(2);int32(2)]')  MultiplexTypes=str2num('[int32(1);int32(1);int32(1);int32(1);int32(1);int32(1);int32(1);int32(1);int32(1);int32(1)]')  MultiplexValues=str2num('[double(0);double(0);double(0);double(0);double(0);double(0);double(0);double(0);double(0);double(0)]')  Factors=str2num('[double(1);double(4);double(4);double(1);double(1);double(1);double(1);double(1);double(1);double(1)]')  Offsets=str2num('[double(0);double(0);double(0);double(-15000);double(-5000);double(0);double(0);double(0);double(0);double(0)]')  Minimums=str2num('[double(-Inf);double(0);double(0);double(-15000);double(-5000);double(-Inf);double(-Inf);double(-Inf);double(-Inf);double(-Inf)]')  Maximums=str2num('[double(Inf);double(16384);double(16384);double(15000);double(5000);double(Inf);double(Inf);double(Inf);double(Inf);double(Inf)]')  Remote=off  ApplyMinMax=off  BusOutput=on
      settings: SourceProductName=Simulink Real-Time  SourceProductBaseCode=XP  DataFormat=CANdb specified signals
  wires:
  ISG HCU Command/1 -> Bus Selector/1
  Bus Selector/2 -> FCAN_Send_ID_0xCFF06EF/2  "<Length>"
  Bus Selector/1 -> FCAN_Send_ID_0xCFF06EF/1  "<Data>"

== system ZT_VehCtrl_18B/SigOut/MCU ==
  "MCU_OUT " : Inport
  Trigger : TriggerPort  VariantControl=Variant  PortDimensions=1
  Bus Selector : BusSelector  OutputSignals=Data,Length
  Bus Selector1 : BusSelector  OutputSignals=Data,Length
  FCAN_Send_ID_0x0C31EFD0 : mbd_mpc574x_ec_toolbox/Communication Blocks/CAN Blocks/FCAN_Send  Priority=2  can_instance=1  can_mode=Non-blocking  can_timeout_ms=0  can_mb_idx=43  can_extended_id=on  can_is_remote=off  can_id=0C31EFD0  show_adv_opts=off  can_fd_enable=off  can_enable_brs=off  can_fd_padding=0
      settings: SourceProductName=NXP Model-Based Design Toolbox for MPC57xx MCUs
  FCAN_Send_ID_0x0C31F1D0 : mbd_mpc574x_ec_toolbox/Communication Blocks/CAN Blocks/FCAN_Send  Priority=2  can_instance=1  can_mode=Non-blocking  can_timeout_ms=0  can_mb_idx=43  can_extended_id=on  can_is_remote=off  can_id=0C31F1D0  show_adv_opts=off  can_fd_enable=off  can_enable_brs=off  can_fd_padding=0
      settings: SourceProductName=NXP Model-Based Design Toolbox for MPC57xx MCUs
  VCU2MCU1 : canmsglib/CAN Pack  CANdbFile=D:\VCU\VCU_SL_ZhengZhou\ZT2\模型与接口\CAN_DBC\动力CANB_GBK.dbc  MsgList=VCU2MCU1  MsgName=VCU2MCU1  MsgIDType=Extended (29-bit identifier)  MsgIdentifier=204599248  MsgLength=8  SignalInfo=VCU2OilMotor_ActiveDisCharge$5$1$1$2$1$0$1$0$0$1$#VCU2OilMotor_AntiSlipEn$4$1$1$2$1$0$1$0$0$1$#VCU2OilMotor_BusCurLimit$8$8$1$2$1$0$4$0$0$1000$#VCU2OilMotor_CtrlBusCounter$56$8$1$2$1$0$1$0$0$255$#VCU2OilMotor_CtrlMode$3$1$1$2$1$0$1$0$0$1$#VCU2OilMotor_En$0$1$1$2$1$0$1$0$0$1$#VCU2OilMotor_RegenVoltLimit$48$8$1$2$1$0$4$0$0$255$#VCU2OilMotor_TarSpd$16$16$1$2$1$0$2.500000e-01$0$0$1.638375e+04$#VCU2OilMotor_TarTrq$32$16$1$2$1$0$1.000000e-01$0$0$6.553500e+03$#VCU2OilMotor_WorkMode$1$2$1$2$1$0$1$0$0$3$#  NSignals=10  StartBits=str2num('[int32(5);int32(4);int32(8);int32(56);int32(3);int32(0);int32(48);int32(16);int32(32);int32(1)]')  SignalSizes=str2num('[int32(1);int32(1);int32(8);int32(8);int32(1);int32(1);int32(8);int32(16);int32(16);int32(2)]')  ByteOrders=str2num('[int32(1);int32(1);int32(1);int32(1);int32(1);int32(1);int32(1);int32(1);int32(1);int32(1)]')  DataTypes=str2num('[int32(2);int32(2);int32(2);int32(2);int32(2);int32(2);int32(2);int32(2);int32(2);int32(2)]')  MultiplexTypes=str2num('[int32(1);int32(1);int32(1);int32(1);int32(1);int32(1);int32(1);int32(1);int32(1);int32(1)]')  MultiplexValues=str2num('[double(0);double(0);double(0);double(0);double(0);double(0);double(0);double(0);double(0);double(0)]')  Factors=str2num('[double(1);double(1);double(4);double(1);double(1);double(1);double(4);double(2.500000e-01);double(1.000000e-01);double(1)]')  Offsets=str2num('[double(0);double(0);double(0);double(0);double(0);double(0);double(0);double(0);double(0);double(0)]')  Minimums=str2num('[double(0);double(0);double(0);double(0);double(0);double(0);double(0);double(0);double(0);double(0)]')  Maximums=str2num('[double(1);double(1);double(1000);double(255);double(1);double(1);double(255);double(1.638375e+04);double(6.553500e+03);double(3)]')  Remote=off  ApplyMinMax=off  BusOutput=on
      settings: SourceProductName=Simulink Real-Time  SourceProductBaseCode=XP  DataFormat=CANdb specified signals
  VCU2MCU2 : canmsglib/CAN Pack  CANdbFile=D:\VCU\VCU_SL_ZhengZhou\ZT2\模型与接口\CAN_DBC\动力CANB_GBK.dbc  MsgList=VCU2MCU2  MsgName=VCU2MCU2  MsgIDType=Extended (29-bit identifier)  MsgIdentifier=204599760  MsgLength=8  SignalInfo=VCU2DrvMotor_ActiveDisCharge$5$1$1$2$1$0$1$0$0$1$#VCU2DrvMotor_AntiSlipEn$4$1$1$2$1$0$1$0$0$1$#VCU2DrvMotor_BusCurLimit$8$8$1$2$1$0$4$0$0$1000$#VCU2DrvMotor_CtrlBusCounter$56$8$1$2$1$0$1$0$0$255$#VCU2DrvMotor_CtrlMode$3$1$1$2$1$0$1$0$0$1$#VCU2DrvMotor_En$0$1$1$2$1$0$1$0$0$1$#VCU2DrvMotor_RegenVoltLimit$48$8$1$2$1$0$4$0$0$255$#VCU2DrvMotor_TarSpd$16$16$1$2$1$0$2.500000e-01$0$0$1.638375e+04$#VCU2DrvMotor_TarTrq$32$16$1$2$1$0$1.000000e-01$0$0$6.553500e+03$#VCU2DrvMotor_WorkMode$1$2$1$2$1$0$1$0$0$3$#  NSignals=10  StartBits=str2num('[int32(5);int32(4);int32(8);int32(56);int32(3);int32(0);int32(48);int32(16);int32(32);int32(1)]')  SignalSizes=str2num('[int32(1);int32(1);int32(8);int32(8);int32(1);int32(1);int32(8);int32(16);int32(16);int32(2)]')  ByteOrders=str2num('[int32(1);int32(1);int32(1);int32(1);int32(1);int32(1);int32(1);int32(1);int32(1);int32(1)]')  DataTypes=str2num('[int32(2);int32(2);int32(2);int32(2);int32(2);int32(2);int32(2);int32(2);int32(2);int32(2)]')  MultiplexTypes=str2num('[int32(1);int32(1);int32(1);int32(1);int32(1);int32(1);int32(1);int32(1);int32(1);int32(1)]')  MultiplexValues=str2num('[double(0);double(0);double(0);double(0);double(0);double(0);double(0);double(0);double(0);double(0)]')  Factors=str2num('[double(1);double(1);double(4);double(1);double(1);double(1);double(4);double(2.500000e-01);double(1.000000e-01);double(1)]')  Offsets=str2num('[double(0);double(0);double(0);double(0);double(0);double(0);double(0);double(0);double(0);double(0)]')  Minimums=str2num('[double(0);double(0);double(0);double(0);double(0);double(0);double(0);double(0);double(0);double(0)]')  Maximums=str2num('[double(1);double(1);double(1000);double(255);double(1);double(1);double(255);double(1.638375e+04);double(6.553500e+03);double(3)]')  Remote=off  ApplyMinMax=off  BusOutput=on
      settings: SourceProductName=Simulink Real-Time  SourceProductBaseCode=XP  DataFormat=CANdb specified signals
  wires:
  VCU2MCU1/1 -> Bus Selector/1
  Bus Selector/2 -> FCAN_Send_ID_0x0C31EFD0/2  "<Length>"
  Bus Selector/1 -> FCAN_Send_ID_0x0C31EFD0/1  "<Data>"
  Bus Selector1/1 -> FCAN_Send_ID_0x0C31F1D0/1  "<Data>"
  Bus Selector1/2 -> FCAN_Send_ID_0x0C31F1D0/2  "<Length>"
  VCU2MCU2/1 -> Bus Selector1/1

== system ZT_VehCtrl_18B/SigOut/PDU ==
  "PDU_OUT " : Inport
  Trigger : TriggerPort  VariantControl=Variant  PortDimensions=1
  Bus Selector : BusSelector  OutputSignals=Data,Length
  FCAN_Send_ID_0x0CF2503B : mbd_mpc574x_ec_toolbox/Communication Blocks/CAN Blocks/FCAN_Send  Priority=2  can_instance=1  can_mode=Non-blocking  can_timeout_ms=0  can_mb_idx=43  can_extended_id=on  can_is_remote=off  can_id=0CF2503B  show_adv_opts=off  can_fd_enable=off  can_enable_brs=off  can_fd_padding=0
      settings: SourceProductName=NXP Model-Based Design Toolbox for MPC57xx MCUs
  VCU_PDU : canmsglib/CAN Pack  CANdbFile=D:\VCU\VCU_SL_ZhengZhou\ZT2\模型与接口\CAN_DBC\动力CANB_GBK.dbc  MsgList=VCU_PDU  MsgName=VCU_PDU  MsgIDType=Extended (29-bit identifier)  MsgIdentifier=217206843  MsgLength=8  SignalInfo=VCU_DCCpstRlyCtl$40$2$1$2$1$0$1$0$-Inf$Inf$#VCU_HVACRlyCtl$6$2$1$2$1$0$1$0$-Inf$Inf$#VCU_HghVtgCnt$16$2$1$2$1$0$1$0$-Inf$Inf$#VCU_HrtBt$56$8$1$2$1$0$1$0$-Inf$Inf$#VCU_PTCRlyCtl$8$2$1$2$1$0$1$0$-Inf$Inf$#VCU_ShrRlyCtl$0$2$1$2$1$0$1$0$-Inf$Inf$#  NSignals=6  StartBits=str2num('[int32(40);int32(6);int32(16);int32(56);int32(8);int32(0)]')  SignalSizes=str2num('[int32(2);int32(2);int32(2);int32(8);int32(2);int32(2)]')  ByteOrders=str2num('[int32(1);int32(1);int32(1);int32(1);int32(1);int32(1)]')  DataTypes=str2num('[int32(2);int32(2);int32(2);int32(2);int32(2);int32(2)]')  MultiplexTypes=str2num('[int32(1);int32(1);int32(1);int32(1);int32(1);int32(1)]')  MultiplexValues=str2num('[double(0);double(0);double(0);double(0);double(0);double(0)]')  Factors=str2num('[double(1);double(1);double(1);double(1);double(1);double(1)]')  Offsets=str2num('[double(0);double(0);double(0);double(0);double(0);double(0)]')  Minimums=str2num('[double(-Inf);double(-Inf);double(-Inf);double(-Inf);double(-Inf);double(-Inf)]')  Maximums=str2num('[double(Inf);double(Inf);double(Inf);double(Inf);double(Inf);double(Inf)]')  Remote=off  ApplyMinMax=off  BusOutput=on
      settings: SourceProductName=Simulink Real-Time  SourceProductBaseCode=XP  DataFormat=CANdb specified signals
  wires:
  Bus Selector/1 -> FCAN_Send_ID_0x0CF2503B/1  "<Data>"
  Bus Selector/2 -> FCAN_Send_ID_0x0CF2503B/2  "<Length>"
  VCU_PDU/1 -> Bus Selector/1

== system ZT_VehCtrl_18B/SigOut/TM ==
  "TM_OUT " : Inport
  Trigger : TriggerPort  VariantControl=Variant  PortDimensions=1
  Bus Selector : BusSelector  OutputSignals=Data,Length
  FCAN_Send_ID_0xCFF05EF : mbd_mpc574x_ec_toolbox/Communication Blocks/CAN Blocks/FCAN_Send  Priority=2  can_instance=1  can_mode=Non-blocking  can_timeout_ms=0  can_mb_idx=43  can_extended_id=on  can_is_remote=off  can_id=CFF05EF  show_adv_opts=off  can_fd_enable=off  can_enable_brs=off  can_fd_padding=0
      settings: SourceProductName=NXP Model-Based Design Toolbox for MPC57xx MCUs
  TM HCU Command : canmsglib/CAN Pack  CANdbFile=D:\VCU\VCU_SL_ZhengZhou\ZT2\模型与接口\CAN_DBC\动力CANB_GBK.dbc  MsgList=TM_HCU_Command  MsgName=TM_HCU_Command  MsgIDType=Extended (29-bit identifier)  MsgIdentifier=218039791  MsgLength=8  SignalInfo=Control_Mode$2$2$1$2$1$0$1$0$-Inf$Inf$#Demand_Limit_High_Positive_Value$8$12$1$2$1$0$4$0$0$16384$#Demand_Limit_Low_Negative_Value$20$12$1$2$1$0$4$0$0$16384$#Demand_Speed$48$16$1$2$1$0$1$-15000$-15000$15000$#Demand_Torque$32$16$1$2$1$0$1$-5000$-5000$5000$#Fault_Reset$1$1$1$2$1$0$1$0$-Inf$Inf$#FootBrake$6$1$1$2$1$0$1$0$-Inf$Inf$#Gear$4$2$1$2$1$0$1$0$-Inf$Inf$#HandBrake$7$1$1$2$1$0$1$0$-Inf$Inf$#MCU_Enable$0$1$1$2$1$0$1$0$-Inf$Inf$#  NSignals=10  StartBits=str2num('[int32(2);int32(8);int32(20);int32(48);int32(32);int32(1);int32(6);int32(4);int32(7);int32(0)]')  SignalSizes=str2num('[int32(2);int32(12);int32(12);int32(16);int32(16);int32(1);int32(1);int32(2);int32(1);int32(1)]')  ByteOrders=str2num('[int32(1);int32(1);int32(1);int32(1);int32(1);int32(1);int32(1);int32(1);int32(1);int32(1)]')  DataTypes=str2num('[int32(2);int32(2);int32(2);int32(2);int32(2);int32(2);int32(2);int32(2);int32(2);int32(2)]')  MultiplexTypes=str2num('[int32(1);int32(1);int32(1);int32(1);int32(1);int32(1);int32(1);int32(1);int32(1);int32(1)]')  MultiplexValues=str2num('[double(0);double(0);double(0);double(0);double(0);double(0);double(0);double(0);double(0);double(0)]')  Factors=str2num('[double(1);double(4);double(4);double(1);double(1);double(1);double(1);double(1);double(1);double(1)]')  Offsets=str2num('[double(0);double(0);double(0);double(-15000);double(-5000);double(0);double(0);double(0);double(0);double(0)]')  Minimums=str2num('[double(-Inf);double(0);double(0);double(-15000);double(-5000);double(-Inf);double(-Inf);double(-Inf);double(-Inf);double(-Inf)]')  Maximums=str2num('[double(Inf);double(16384);double(16384);double(15000);double(5000);double(Inf);double(Inf);double(Inf);double(Inf);double(Inf)]')  Remote=off  ApplyMinMax=off  BusOutput=on
      settings: SourceProductName=Simulink Real-Time  SourceProductBaseCode=XP  DataFormat=CANdb specified signals
  wires:
  Bus Selector/1 -> FCAN_Send_ID_0xCFF05EF/1  "<Data>"
  Bus Selector/2 -> FCAN_Send_ID_0xCFF05EF/2  "<Length>"
  TM HCU Command/1 -> Bus Selector/1

== system ZT_VehCtrl_18B/SigOut/TMS1 ==
  "TMS_OUT " : Inport
  Trigger : TriggerPort  VariantControl=Variant  PortDimensions=1
  Bus Selector : BusSelector  OutputSignals=Data,Length
  Constant1 : Constant  Value=8
  Constant2 : Constant  Value=hex2dec('40')
  Constant3 : Constant  Value=hex2dec('04')
  Constant4 : Constant  Value=hex2dec('10')
  Constant5 : Constant  Value=0
  Data Type Conversion : DataTypeConversion
  Data Type Conversion1 : DataTypeConversion
  FCAN_Send_ID_0x18FFF347 : mbd_mpc574x_ec_toolbox/Communication Blocks/CAN Blocks/FCAN_Send  Priority=2  can_instance=0  can_mode=Non-blocking  can_timeout_ms=0  can_mb_idx=45  can_extended_id=on  can_is_remote=off  can_id=18FFF347  show_adv_opts=off  can_fd_enable=off  can_enable_brs=off  can_fd_padding=0
      settings: SourceProductName=NXP Model-Based Design Toolbox for MPC57xx MCUs
  FCAN_Send_ID_0x3FF1 : mbd_mpc574x_ec_toolbox/Communication Blocks/CAN Blocks/FCAN_Send  Priority=2  can_instance=2  can_mode=Non-blocking  can_timeout_ms=0  can_mb_idx=51  can_extended_id=off  can_is_remote=off  can_id=605  show_adv_opts=off  can_fd_enable=off  can_enable_brs=off  can_fd_padding=0
      settings: SourceProductName=NXP Model-Based Design Toolbox for MPC57xx MCUs
  Mux : Mux  Inputs=8
  TMS : canmsglib/CAN Pack  CANdbFile=D:\VCU\VCU_SL_ZhengZhou\ZT2\模型与接口\CAN_DBC\整车CANA_GBK.dbc  MsgList=VCU2TMS  MsgName=VCU2TMS  MsgIDType=Extended (29-bit identifier)  MsgIdentifier=419427143  MsgLength=8  SignalInfo=VCU_FanSpeedLvl_num$0$8$2$2$1$0$1$0$0$255$#VCU_Life1_num$56$8$2$2$1$0$1$0$0$255$#  NSignals=2  StartBits=str2num('[int32(0);int32(56)]')  SignalSizes=str2num('[int32(8);int32(8)]')  ByteOrders=str2num('[int32(2);int32(2)]')  DataTypes=str2num('[int32(2);int32(2)]')  MultiplexTypes=str2num('[int32(1);int32(1)]')  MultiplexValues=str2num('[double(0);double(0)]')  Factors=str2num('[double(1);double(1)]')  Offsets=str2num('[double(0);double(0)]')  Minimums=str2num('[double(0);double(0)]')  Maximums=str2num('[double(255);double(255)]')  Remote=off  ApplyMinMax=off  BusOutput=on
      settings: SourceProductName=Simulink Real-Time  SourceProductBaseCode=XP  DataFormat=CANdb specified signals
  wires:
  Constant2/1 -> Mux/1
  Data Type Conversion/1 -> FCAN_Send_ID_0x3FF1/1
  Constant5/1 -> Mux/4, Mux/7, Mux/8, Mux/6, Mux/5
  Data Type Conversion1/1 -> FCAN_Send_ID_0x3FF1/2
  Constant1/1 -> Data Type Conversion1/1
  Mux/1 -> Data Type Conversion/1
  Constant3/1 -> Mux/2
  Constant4/1 -> Mux/3
  TMS/1 -> Bus Selector/1
  Bus Selector/1 -> FCAN_Send_ID_0x18FFF347/1  "<Data>"
  Bus Selector/2 -> FCAN_Send_ID_0x18FFF347/2  "<Length>"

== system ZT_VehCtrl_18B/SigOut/TWV ==
  "TWV_OUT " : Inport
  Trigger : TriggerPort  VariantControl=Variant  PortDimensions=1
  Bus Selector : BusSelector  OutputSignals=Data,Length
  FCAN_Send_ID_0x18FF25EF : mbd_mpc574x_ec_toolbox/Communication Blocks/CAN Blocks/FCAN_Send  Priority=2  can_instance=1  can_mode=Non-blocking  can_timeout_ms=0  can_mb_idx=43  can_extended_id=on  can_is_remote=off  can_id=18FF25EF  show_adv_opts=off  can_fd_enable=off  can_enable_brs=off  can_fd_padding=0
      settings: SourceProductName=NXP Model-Based Design Toolbox for MPC57xx MCUs
  VCU_TWV : canmsglib/CAN Pack  CANdbFile=D:\VCU\VCU_SL_ZhengZhou\ZT2\模型与接口\CAN_DBC\动力CANB_GBK.dbc  MsgList=VCU_TWV  MsgName=VCU_TWV  MsgIDType=Extended (29-bit identifier)  MsgIdentifier=419374575  MsgLength=8  SignalInfo=VCU_TWV1_P_MoveEnable$33$1$1$2$1$0$1$0$0$1$#VCU_TWV1_P_PosSet$24$8$1$2$1$0$4.000000e-01$0$0$100$#  NSignals=2  StartBits=str2num('[int32(33);int32(24)]')  SignalSizes=str2num('[int32(1);int32(8)]')  ByteOrders=str2num('[int32(1);int32(1)]')  DataTypes=str2num('[int32(2);int32(2)]')  MultiplexTypes=str2num('[int32(1);int32(1)]')  MultiplexValues=str2num('[double(0);double(0)]')  Factors=str2num('[double(1);double(4.000000e-01)]')  Offsets=str2num('[double(0);double(0)]')  Minimums=str2num('[double(0);double(0)]')  Maximums=str2num('[double(1);double(100)]')  Remote=off  ApplyMinMax=off  BusOutput=on
      settings: SourceProductName=Simulink Real-Time  SourceProductBaseCode=XP  DataFormat=CANdb specified signals
  wires:
  VCU_TWV/1 -> Bus Selector/1
  Bus Selector/2 -> FCAN_Send_ID_0x18FF25EF/2  "<Length>"
  Bus Selector/1 -> FCAN_Send_ID_0x18FF25EF/1  "<Data>"
